simulink model "charging"  (R2022b)
settings: Solver=VariableStepAuto  StartTime=0.0  StopTime=10.0  RelTol=1e-3
libraries: fl_lib x7, ee_lib x5, nesl_utility x4, batteryecm_lib x1
settings Model: Creator=minar  LastModifiedBy=minar

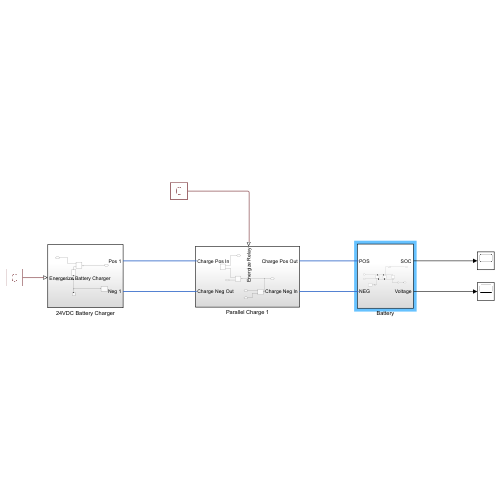
[thumbnail: Simulink's stored preview of the top-level diagram]
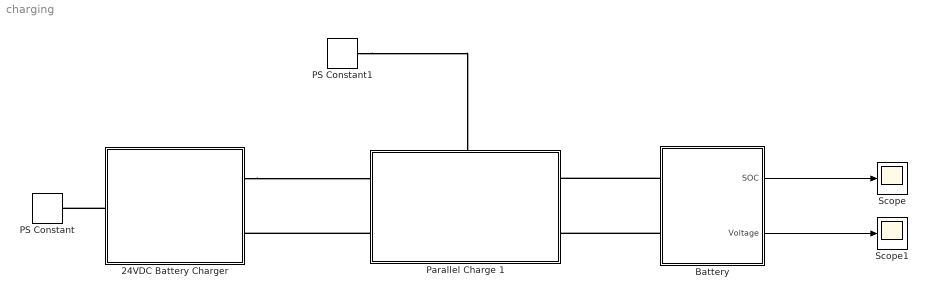
== system charging ==
  24VDC Battery Charger : Subsystem
  Battery : Subsystem
  PS Constant : fl_lib/Physical Signals/Sources/PS Constant  constant=1
  PS Constant1 : fl_lib/Physical Signals/Sources/PS Constant  constant=1
  Parallel Charge 1 : Subsystem
      settings: PortSchema="{\"entries\":[{\"content\":{\"sides\":[{\"content\":{\"connectorIds\":[\"LConn1\",\"LConn2\"]},\"type\":\"ConnectorPlacement.EquallySpacedRectSide\",\"uuid\":\"92b66880-3ab5-48ec-aaf6-0b390f6e8e6c\"},{\"content\":{\"connectorIds\":[\"RConn1\",\"RConn2\"],\"side\":\"RIGHT\"},\"type\":\"ConnectorPlacement.EquallySpacedRectSide\",\"uuid\":\"e85905ce-1804-41fb-a21c-30ce2b9855cf\"},{\"content\":{\"connectorIds\":[\"LConn3\"],\"side\":\"TOP\"},\"type\":\"ConnectorPlacement.EquallySpacedRectSide\",\"uuid\":\"eff338fa-75bd-4848-9daa-8afb385e699a\"}]},\"type\":\"ConnectorPlacement.EquallySpacedConnector\",\"uuid\":\"4f6beb8f-1b0c-4e7d-9e2e-53f134c38bf2\"}],\"packageUris\":[\"http://schema.mathworks.com/mf0/Connector/R2020b\"],\"version\":\"1.0\"}"
  Scope : Scope
  Scope1 : Scope
  wires:
  Battery/2(Voltage) -> Scope1/1
  Battery/1(SOC) -> Scope/1
  connections:
  24VDC Battery Charger/RConn1 -- PS Constant/RConn1
  24VDC Battery Charger/LConn1 -- Parallel Charge 1/LConn1
  Parallel Charge 1/LConn2 -- 24VDC Battery Charger/LConn2
  PS Constant1/RConn1 -- Parallel Charge 1/LConn3
  Battery/LConn1 -- Parallel Charge 1/RConn1
  Battery/LConn2 -- Parallel Charge 1/RConn2

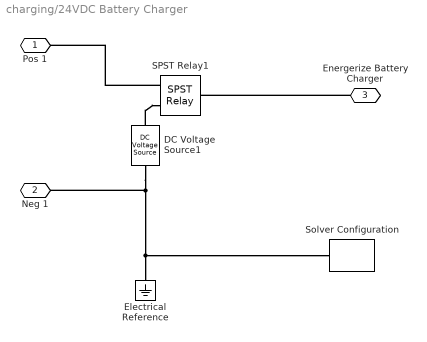
== system charging/24VDC Battery Charger ==
  DC Voltage Source1 : fl_lib/Electrical/Electrical Sources/DC Voltage Source  v0=24 V
  Electrical Reference : fl_lib/Electrical/Electrical Elements/Electrical Reference
  SPST Relay1 : ee_lib/Switches & Breakers/Relays/SPST Relay  block_choices=ee.enum.controlport.ps  R_closed=0.01 Ohm  G_open=1e-8 1/Ohm  Threshold=1  exposemeasurement=ee.enum.exposemeasurement.hidden  V_rated=5 V  V_energize=75  V_deenergize=25  l_winding=0.08 H  r_winding=12.5 Ohm  g_winding=1e-9 1/Ohm  T_brk_C_S=0 s  T_mak_C_S=0 s  enable_faults=ee.enum.relays.enable.no  fault_action=ee.enum.relays.faultaction.none  fault_types=ee.enum.relays.faultTypes.winding  fault_condition_ps=ee.enum.relays.faultConditionSPSTps.csstuck  r_deg_closed_s=1e-9 Ohm  winding_tau_fault=1e-3 s  tau_fault=1e-3 s  enable_temporal_fault=ee.enum.relays.enable.no  t_fault_stick=1 s  t_fault_ComOpen=1 s  t_fault=1 s  enable_behavioral_fault=ee.enum.relays.enable.no  winding_max_permissible_voltage=inf V  n_fail_on_voltage=1  winding_max_permissible_current=inf A  max_permissible_current=inf A  t_fail_on_current=1 s
      settings: InternalSimscapePortConfiguration="{\"Bottom\":[],\"Left\":[{\"id\":\"PS\",\"label\":\"PS\",\"type\":\"input\"}],\"Right\":[{\"id\":\"S\",\"label\":\"S\",\"type\":\"foundation.electrical.electrical\"},{\"id\":\"COM\",\"label\":\"C\",\"type\":\"foundation.electrical.electrical\"}],\"Top\":[]}"
  Solver Configuration : nesl_utility/Solver Configuration  PhysicalDomain=network_engine_domain  SubClassName=solver  LeftPortType=input  RightPortType=generic  Tones=[]  Harmonics=[]  SimulateNoise=off  Profile=off  UseLocalSampling=off  EnableSwitchedLinearOptims=on  FrequencyDomain=off  UseCCode=off  RelTol=0.001  AbsTol=0.001  MinStep=1e-09  ToWorkspace=off  RevertToSquareIcSolve=off  NumHomotopyIterations=100  PhasorMode=off  PhasorModeNumHarmonics=1  ConsistencySolver=NEWTON_XTOL_AFTER_FTOL  IndexReductionMethod=DerivativeReplacement  DoDC=off  ResidualTolerance=1e-09  ConsistencyTolSource=GLOBAL  ConsistencyAbsTol=0.001  ConsistencyRelTol=0.001  ConsistencyTolFactor=0.001  UseLocalSolver=off  LocalSolverChoice=NE_BACKWARD_EULER_ADVANCER  ResolveIndetEquations=on  FunctionEvalNumThread=1  LocalSolverSampleTime=0.001  DoFixedCost=off  MaxNonlinIter=3  MaxModeIter=2  ComputeImpulses=off  ImpulseIterations=2  LinearAlgebra=auto  LinearAlgebraNumThread=0  EquationFormulation=NE_TIME_EF  DelaysMemoryBudget=1024  AutomaticFiltering=on  FilteringTimeConstant=0.001  PartitionStorageMethod=AS_NEEDED  PartitionMemoryBudget=1024  PartitionMethod=ROBUST
  Pos 1 : PMIOPort  Side=Left
  Neg 1 : PMIOPort  Port=2  Side=Left
  Energerize Battery Charger : PMIOPort  Port=3  Side=Right
  connections:
  Energerize Battery Charger/RConn1 -- SPST Relay1/LConn1
  SPST Relay1/RConn2 -- Pos 1/RConn1
  DC Voltage Source1/RConn1 -- Neg 1/RConn1 -- Solver Configuration/RConn1 -- Electrical Reference/LConn1
  DC Voltage Source1/LConn1 -- SPST Relay1/RConn1

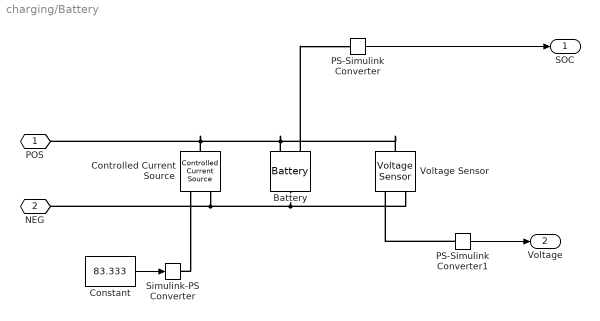
== system charging/Battery ==
  Battery : batteryecm_lib/Battery  Vnom=2.2 V  prm_dir=simscape.enum.battery.prm_dir.disabled  R1_dis=2 Ohm  R1_ch=2 Ohm  R1=2 Ohm  prm_AH=simscape.enum.battery.prm_AH.finite  AH=11573.9 A*hr  V1=1 V  AH1=11396 A*hr  prm_R2=simscape.enum.battery.prm_R2.disabled  R2=2000 Ohm  prm_dyn=simscape.enum.battery.prm_dyn.off  Rp1=0.005 Ohm  tau1=30 s  Rp2=0.005 Ohm  tau2=30 s  Rp3=0.005 Ohm  tau3=30 s  Rp4=0.005 Ohm  tau4=30 s  Rp5=0.005 Ohm  tau5=30 s  prm_fade=simscape.enum.battery.prm_fade.disabled  N_fade=100  AH_fade=45 A*hr  R1_fade=2.02 Ohm  R1_ch_fade=2.02 Ohm  V1_fade=10.35 V  prm_age=simscape.enum.battery.prm_age.disabled  prm_age_OCV=simscape.enum.battery.prm_age_OCV.OCV  OCV_age=0.9  SOC_age=60  delta_time_age_vec=[0] d  temperature_age_vec=[273] K  OCV_scaling_age=2.2134e6  OCV_offset_age=1.632e6  temp_exp_age=0.515833569 V  t_exp_age=0.75  i_specify=off  i_priority=None  i=0 A  i_nominal_specify=off  i_nominal_unit=A  i_nominal_value=1  v_specify=off  v_priority=None  v=0 V  v_nominal_specify=off  v_nominal_unit=V  v_nominal_value=2.2  charge_specify=off  charge_priority=High  charge=50 A*hr  charge_nominal_specify=off  charge_nominal_unit=A*hr  charge_nominal_value=1  num_cycles_specify=off  num_cycles_priority=High  num_cycles=0  num_cycles_nominal_specify=off  num_cycles_nominal_unit=1  num_cycles_nominal_value=1  Tmeas=298.15 K  Tmeas_age=298.15 K  Vnom_T2=12 V  R1_T2=2.2 Ohm  R1_T2_dis=2.2 Ohm  R1_T2_ch=2.2 Ohm  V1_T2=11.4 V  R2_T2=2200 Ohm  Rp1_T2=0.005 Ohm  tau1_T2=30 s  Rp2_T2=0.005 Ohm  tau2_T2=30 s  Rp3_T2=0.005 Ohm  tau3_T2=30 s  Rp4_T2=0.005 Ohm  tau4_T2=30 s  Rp5_T2=0.005 Ohm  tau5_T2=30 s  Tmeas2=273.15 K  thermal_mass=30000 J/K  temperature_specify=off  temperature_priority=High  temperature=298.15 K  temperature_nominal_specify=off  temperature_nominal_unit=K  temperature_nominal_value=1
      settings: InternalSimscapePortConfiguration="{\"Bottom\":[],\"Left\":[{\"id\":\"p\",\"label\":\"+\",\"type\":\"foundation.electrical.electrical\"},{\"id\":\"q\",\"label\":\"q\",\"type\":\"output\"}],\"Right\":[{\"id\":\"n\",\"label\":\"-\",\"type\":\"foundation.electrical.electrical\"}],\"Top\":[]}"
  Constant : Constant  Value=83.333
  Controlled Current Source : fl_lib/Electrical/Electrical Sources/Controlled Current Source
  PS-Simulink Converter : nesl_utility/PS-Simulink Converter  PhysicalDomain=network_engine_domain  SubClassName=ps_output  LeftPortType=input  RightPortType=output  PseudoPeriodic=off  Frequencies=[]  VectorFormat=inherit  Unit=inherit  AffineConversion=off
  PS-Simulink Converter1 : nesl_utility/PS-Simulink Converter  PhysicalDomain=network_engine_domain  SubClassName=ps_output  LeftPortType=input  RightPortType=output  PseudoPeriodic=off  Frequencies=[]  VectorFormat=inherit  Unit=inherit  AffineConversion=off
  Simulink-PS Converter : nesl_utility/Simulink-PS Converter  PhysicalDomain=network_engine_domain  SubClassName=ps_input  LeftPortType=input  RightPortType=output  PseudoPeriodic=off  Frequencies=[]  NoiseDistribution=none  NoiseParameters=[]  Unit=1  AffineConversion=off  FilteringAndDerivatives=provide  SimscapeFilterOrder=1  InputFilterTimeConstant=0.001  UdotUserProvided=0
  Voltage Sensor : fl_lib/Electrical/Electrical Sensors/Voltage Sensor
  POS : PMIOPort  Side=Left
  NEG : PMIOPort  Port=2  Side=Left
  SOC : Outport
  Voltage : Outport  Port=2
  wires:
  Constant/1 -> Simulink-PS Converter/1
  PS-Simulink Converter/1 -> SOC/1
  PS-Simulink Converter1/1 -> Voltage/1
  connections:
  Battery/LConn2 -- PS-Simulink Converter/LConn1
  PS-Simulink Converter1/LConn1 -- Voltage Sensor/RConn1
  Voltage Sensor/LConn1 -- Battery/LConn1 -- Controlled Current Source/LConn1 -- POS/RConn1
  Voltage Sensor/RConn2 -- Battery/RConn1 -- Controlled Current Source/RConn2 -- NEG/RConn1
  Controlled Current Source/RConn1 -- Simulink-PS Converter/RConn1

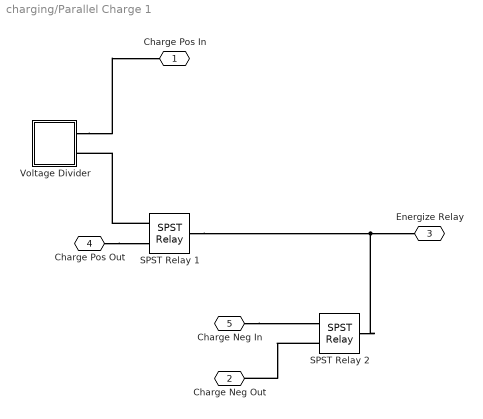
== system charging/Parallel Charge 1 ==
  SPST Relay 1 : ee_lib/Switches & Breakers/Relays/SPST Relay  block_choices=ee.enum.controlport.ps  R_closed=0.01 Ohm  G_open=1e-8 1/Ohm  Threshold=1  exposemeasurement=ee.enum.exposemeasurement.hidden  V_rated=5 V  V_energize=75  V_deenergize=25  l_winding=0.08 H  r_winding=12.5 Ohm  g_winding=1e-9 1/Ohm  T_brk_C_S=0 s  T_mak_C_S=0 s  enable_faults=ee.enum.relays.enable.no  fault_action=ee.enum.relays.faultaction.none  fault_types=ee.enum.relays.faultTypes.winding  fault_condition_ps=ee.enum.relays.faultConditionSPSTps.csstuck  r_deg_closed_s=1e-9 Ohm  winding_tau_fault=1e-3 s  tau_fault=1e-3 s  enable_temporal_fault=ee.enum.relays.enable.no  t_fault_stick=1 s  t_fault_ComOpen=1 s  t_fault=1 s  enable_behavioral_fault=ee.enum.relays.enable.no  winding_max_permissible_voltage=inf V  n_fail_on_voltage=1  winding_max_permissible_current=inf A  max_permissible_current=inf A  t_fail_on_current=1 s
      settings: InternalSimscapePortConfiguration="{\"Bottom\":[],\"Left\":[{\"id\":\"PS\",\"label\":\"PS\",\"type\":\"input\"}],\"Right\":[{\"id\":\"S\",\"label\":\"S\",\"type\":\"foundation.electrical.electrical\"},{\"id\":\"COM\",\"label\":\"C\",\"type\":\"foundation.electrical.electrical\"}],\"Top\":[]}"
  SPST Relay 2 : ee_lib/Switches & Breakers/Relays/SPST Relay  block_choices=ee.enum.controlport.ps  R_closed=0.01 Ohm  G_open=1e-8 1/Ohm  Threshold=1  exposemeasurement=ee.enum.exposemeasurement.hidden  V_rated=5 V  V_energize=75  V_deenergize=25  l_winding=0.08 H  r_winding=12.5 Ohm  g_winding=1e-9 1/Ohm  T_brk_C_S=0 s  T_mak_C_S=0 s  enable_faults=ee.enum.relays.enable.no  fault_action=ee.enum.relays.faultaction.none  fault_types=ee.enum.relays.faultTypes.winding  fault_condition_ps=ee.enum.relays.faultConditionSPSTps.csstuck  r_deg_closed_s=1e-9 Ohm  winding_tau_fault=1e-3 s  tau_fault=1e-3 s  enable_temporal_fault=ee.enum.relays.enable.no  t_fault_stick=1 s  t_fault_ComOpen=1 s  t_fault=1 s  enable_behavioral_fault=ee.enum.relays.enable.no  winding_max_permissible_voltage=inf V  n_fail_on_voltage=1  winding_max_permissible_current=inf A  max_permissible_current=inf A  t_fail_on_current=1 s
      settings: InternalSimscapePortConfiguration="{\"Bottom\":[],\"Left\":[{\"id\":\"PS\",\"label\":\"PS\",\"type\":\"input\"}],\"Right\":[{\"id\":\"S\",\"label\":\"S\",\"type\":\"foundation.electrical.electrical\"},{\"id\":\"COM\",\"label\":\"C\",\"type\":\"foundation.electrical.electrical\"}],\"Top\":[]}"
  Voltage Divider : Subsystem
  Charge Pos In : PMIOPort  Side=Left
  Charge Neg Out : PMIOPort  Port=2  Side=Left
  Energize Relay : PMIOPort  Port=3  Side=Left
  Charge Pos Out : PMIOPort  Port=4  Side=Right
  Charge Neg In : PMIOPort  Port=5  Side=Right
  connections:
  SPST Relay 2/RConn2 -- Charge Neg Out/RConn1
  Charge Neg In/RConn1 -- SPST Relay 2/RConn1
  Charge Pos Out/RConn1 -- SPST Relay 1/RConn2
  SPST Relay 1/LConn1 -- Energize Relay/RConn1 -- SPST Relay 2/LConn1
  Voltage Divider/RConn1 -- Charge Pos In/RConn1
  SPST Relay 1/RConn1 -- Voltage Divider/RConn2

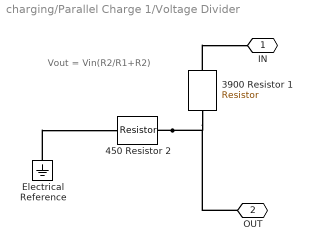
== system charging/Parallel Charge 1/Voltage Divider ==
  note: Vout = Vin(R2/R1+R2)
  3900 Resistor 1 : ee_lib/Passive/Resistor  R=3900 Ohm  enable_R_tol=0  R_tol=5  tol_distribution=1  nSigma=4  enable_operating_limits=0  operating_limit_action=2  max_working_voltage=100 V  power_rating=1 W  enable_faults=0  fault_action=1  R_faulted=inf Ohm  enable_temporal_fault=0  t_fault=1 s  enable_behavioral_fault=0  max_permissible_current=1 A  t_fail_on_current=1 s  noise_mode=0  sample_time=1e-3 s  repeatability=1  auto_seed=3499211588  user_seed=0  Tdevice=25 degC  power_derating_T1=70 degC  power_derating_T2=155 degC  operating_temperature_range_vec=[-50, 150] degC  alpha=3.93e-3 1/K  Tmeas=25 degC  thermal_mass=100 J/K  temperature_specify=off  temperature_priority=High  temperature=298.15 K  temperature_nominal_specify=off  temperature_nominal_unit=K  temperature_nominal_value=1
  450 Resistor 2 : ee_lib/Passive/Resistor  R=450 Ohm  enable_R_tol=0  R_tol=5  tol_distribution=1  nSigma=4  enable_operating_limits=0  operating_limit_action=2  max_working_voltage=100 V  power_rating=1 W  enable_faults=0  fault_action=1  R_faulted=inf Ohm  enable_temporal_fault=0  t_fault=1 s  enable_behavioral_fault=0  max_permissible_current=1 A  t_fail_on_current=1 s  noise_mode=0  sample_time=1e-3 s  repeatability=1  auto_seed=3890346746  user_seed=0  Tdevice=25 degC  power_derating_T1=70 degC  power_derating_T2=155 degC  operating_temperature_range_vec=[-50, 150] degC  alpha=3.93e-3 1/K  Tmeas=25 degC  thermal_mass=100 J/K  temperature_specify=off  temperature_priority=High  temperature=298.15 K  temperature_nominal_specify=off  temperature_nominal_unit=K  temperature_nominal_value=1
  Electrical Reference : fl_lib/Electrical/Electrical Elements/Electrical Reference
  IN : PMIOPort  Side=Right
  OUT : PMIOPort  Port=2  Side=Right
  connections:
  450 Resistor 2/LConn1 -- OUT/RConn1 -- 3900 Resistor 1/LConn1
  3900 Resistor 1/RConn1 -- IN/RConn1
  Electrical Reference/LConn1 -- 450 Resistor 2/RConn1
